simulink model "BSPD_Gradient"  (R2016b)
settings: Solver=ode23tb  StartTime=0.0  StopTime=1000  RelTol=1e-3
settings Model: Creator=Niels  LastModifiedBy=Niels
settings SolverCC: ZeroCrossAlgorithm=Adaptive

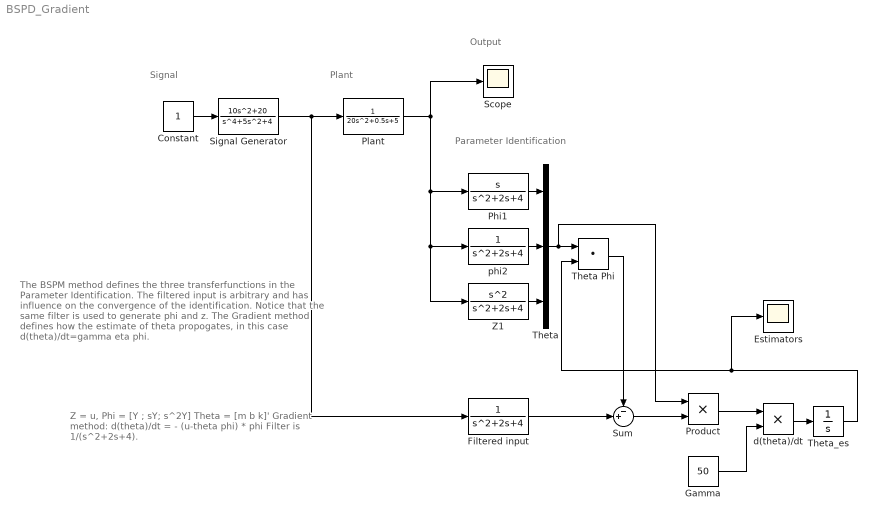
== system BSPD_Gradient ==
  note: Z = u,
      | Phi = [Y ; sY; s^2Y]
      | Theta = [m b k]'
      | Gradient method: d(theta)/dt = - (u-theta phi) * phi
      | Filter is 1/(s^2+2s+4).
  note: The BSPM method defines the three transferfunctions in the
      | Parameter Identification. The filtered input is arbitrary and has
      | influence on the convergence of the identification. Notice that
      | the same filter is used to generate phi and z.
      | The Gradient method defines how the estimate of theta
      | propogates, in this case d(theta)/dt=gamma eta phi.
  note: Parameter Identification
  note: Output
  note: Plant
  note: Signal
  Constant : Constant
  Estimators : Scope
  "Filtered input " : TransferFcn  Denominator=[1 2 4]
  "Gamma " : Constant  Value=50
  "Phi1 " : TransferFcn  Numerator=[1 0]  Denominator=[1 2 4]
  Plant : TransferFcn  Denominator=[20 0.5 5]
  Product : Product
  Scope : Scope
  Signal Generator : TransferFcn  Numerator=[10 0 20]  Denominator=[1 0 5 0 4]
  Sum : Sum  Inputs=-+|
  Theta : Concatenate  NumInputs=3
  Theta Phi : DotProduct  InputSameDT=on  OutDataTypeStr=Inherit: Inherit via internal rule
  Theta_es : Integrator
  Z1 : TransferFcn  Numerator=[1 0 0]  Denominator=[1 2 4]
  d(theta)/dt : Product
  phi2 : TransferFcn  Denominator=[1 2 4]
  wires:
  Constant/1 -> Signal Generator/1
  Signal Generator/1 -> "Filtered input "/1, Plant/1
  Plant/1 -> "Phi1 "/1, phi2/1, Z1/1, Scope/1
  phi2/1 -> Theta/2
  "Phi1 "/1 -> Theta/1
  Z1/1 -> Theta/3
  Theta/1 -> Product/1, Theta Phi/1
  Theta Phi/1 -> Sum/1
  "Filtered input "/1 -> Sum/2
  Sum/1 -> Product/2
  Product/1 -> d(theta)/dt/1
  "Gamma "/1 -> d(theta)/dt/2
  d(theta)/dt/1 -> Theta_es/1
  Theta_es/1 -> Estimators/1, Theta Phi/2
